simulink model "New_simulation_compare_test"  (R2018b)
settings: Solver=VariableStepAuto  StartTime=0.0  StopTime=10.0  RelTol=1e-3
undefined symbols (not defined in the file or in its folder): DiscIntNeverNeededParam, sigbuilder_block
libraries: commchan3 x2, simulink x2, visionstatistics x1
settings Model: Creator=UWEcocar  LastModifiedBy=UWEcocar

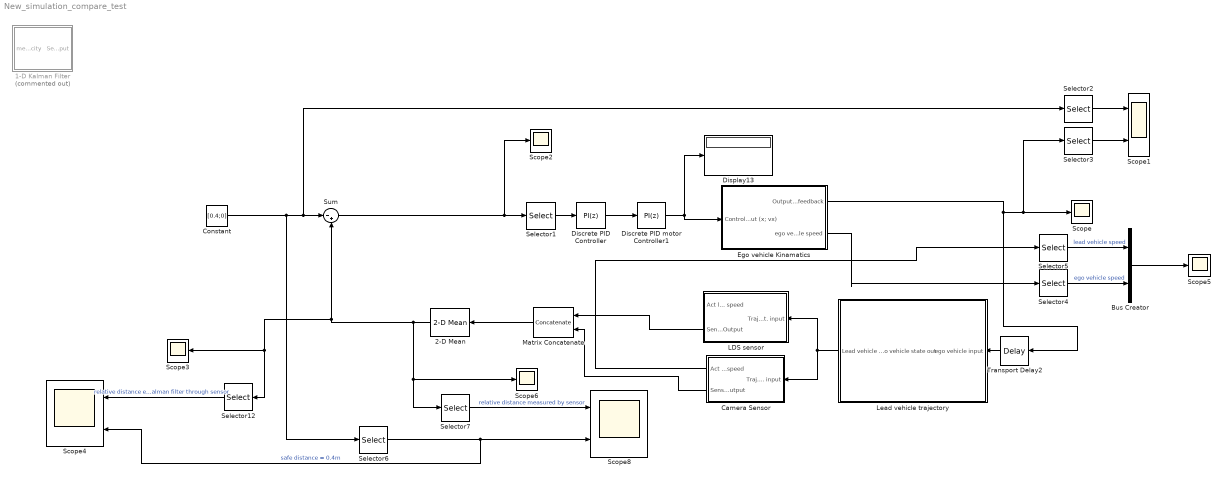
== system New_simulation_compare_test ==
  1-D Kalman Filter : Subsystem  Commented=on
  2-D Mean : visionstatistics/2-D Mean  run=off  reset_popup=None  directionMode=Each row  dimension=1  treatSBRowAsCol=on  roiEnable=off  roiType=Rectangles  roiPortion=Entire ROI  roiOutput=Individual statistics for each ROI  roiFlag=off  outputDataTypeStr=Inherit: Same as accumulator  outputLastDataTypeStr=Inherit: Same as accumulator  outputMin=[]  outputMax=[]  accumMode=Binary point scaling  accumWordLength=32  accumFracLength=0  accumDataTypeStr=fixdt([],32,0)  accumLastDataTypeStr=fixdt([],32,0)  roundingMode=Floor  overflowMode=off
      settings: SourceProductName=Computer Vision System Toolbox  SourceProductBaseCode=VP
  Bus Creator : BusCreator  Inputs=2
  Camera Sensor : Subsystem
  Constant : Constant  Value=[0.4;0]  VectorParams1D=off
  Discrete PID Controller : simulink/Continuous/PID Controller  Controller=PI  Form=Parallel  TimeDomain=Discrete-time  SampleTime=-1  IntegratorMethod=Forward Euler  FilterMethod=Forward Euler  ControllerParametersSource=internal  P=.26  I=.001  D=0  UseFilter=on  N=100  TunerSelectOption=Transfer Function Based (PID Tuner App)  InitialConditionSource=internal  InitialConditionForIntegrator=0  InitialConditionForFilter=0  DifferentiatorICPrevScaledInput=0  ExternalReset=none  TrackingMode=off  Kt=1  LimitOutput=on  UpperSaturationLimit=0.2  LowerSaturationLimit=-0.2  LinearizeAsGain=off  AntiWindupMode=clamping  Kb=1  POutMin=[]  POutMax=[]  IOutMin=[]  IOutMax=[]  DOutMin=[]  DOutMax=[]  NOutMin=[]  NOutMax=[]  SumOutMin=[]  SumOutMax=[]  SaturationOutMin=[]  SaturationOutMax=[]  PParamMin=[]  PParamMax=[]  IParamMin=[]  IParamMax=[]  DParamMin=[]  DParamMax=[]  NParamMin=[]  NParamMax=[]  KbParamMin=[]  KbParamMax=[]  KtParamMin=[]  KtParamMax=[]  KbOutMin=[]  KbOutMax=[]  KtOutMin=[]  KtOutMax=[]  IntegratorOutMin=[]  IntegratorOutMax=[]  FilterOutMin=[]  FilterOutMax=[]  SumI1OutMin=[]  SumI1OutMax=[]  SumI2OutMin=[]  SumI2OutMax=[]  SumI3OutMin=[]  SumI3OutMax=[]  SumI4OutMin=[]  SumI4OutMax=[]  SumDOutMin=[]  SumDOutMax=[]  DifferentiatorOutMin=[]  DifferentiatorOutMax=[]  FilterDiffOutCoefMin=[]  FilterDiffOutCoefMax=[]  ReciprocalOutMin=[]  ReciprocalOutMax=[]  SumDenOutMin=[]  SumDenOutMax=[]  SumNumOutMin=[]  SumNumOutMax=[]  DivideOutMin=[]  DivideOutMax=[]  IntegratorContinuousStateAttributes=''  IntegratorStateMustResolveToSignalObject=off  IntegratorRTWStateStorageClass=Auto  FilterContinuousStateAttributes=''  FilterStateMustResolveToSignalObject=off  FilterRTWStateStorageClass=Auto  ParallelPVariant=InternalParameters  IdealPVariant=Disabled  IVariant=InternalParameters  DVariant=Disabled  IntegratorVariant=Discrete  SatVariant=Enabled  AWVariant=DiscClampingParallel  PCopyVariant=Disabled  TRVariant=Disabled  FdbkBlocksVariant=Forward  IdealPFdbkVariant=Disabled  SatFdbkVariant=Disabled  DerivativeFilterVariant=Disabled  NVariant=Disabled  NCopyVariant=Disabled_SignalSpec  FilterICVariant=Disabled  IntegratorICVariant=InternalICs  ExternalResetVariant=Disabled  TRSumVariant=Passthrough  SumFdbkVariant=Disabled  SumVariant=Sum_PI
  Discrete PID motor Controller1 : simulink/Continuous/PID Controller  Controller=PI  Form=Parallel  TimeDomain=Discrete-time  SampleTime=-1  IntegratorMethod=Forward Euler  FilterMethod=Forward Euler  ControllerParametersSource=internal  P=0.7813  I=0.0153  D=0  UseFilter=on  N=100  TunerSelectOption=Transfer Function Based (PID Tuner App)  InitialConditionSource=internal  InitialConditionForIntegrator=0  InitialConditionForFilter=0  DifferentiatorICPrevScaledInput=0  ExternalReset=none  TrackingMode=off  Kt=1  LimitOutput=on  UpperSaturationLimit=0.2  LowerSaturationLimit=-0.2  LinearizeAsGain=off  AntiWindupMode=clamping  Kb=1  POutMin=[]  POutMax=[]  IOutMin=[]  IOutMax=[]  DOutMin=[]  DOutMax=[]  NOutMin=[]  NOutMax=[]  SumOutMin=[]  SumOutMax=[]  SaturationOutMin=[]  SaturationOutMax=[]  PParamMin=[]  PParamMax=[]  IParamMin=[]  IParamMax=[]  DParamMin=[]  DParamMax=[]  NParamMin=[]  NParamMax=[]  KbParamMin=[]  KbParamMax=[]  KtParamMin=[]  KtParamMax=[]  KbOutMin=[]  KbOutMax=[]  KtOutMin=[]  KtOutMax=[]  IntegratorOutMin=[]  IntegratorOutMax=[]  FilterOutMin=[]  FilterOutMax=[]  SumI1OutMin=[]  SumI1OutMax=[]  SumI2OutMin=[]  SumI2OutMax=[]  SumI3OutMin=[]  SumI3OutMax=[]  SumI4OutMin=[]  SumI4OutMax=[]  SumDOutMin=[]  SumDOutMax=[]  DifferentiatorOutMin=[]  DifferentiatorOutMax=[]  FilterDiffOutCoefMin=[]  FilterDiffOutCoefMax=[]  ReciprocalOutMin=[]  ReciprocalOutMax=[]  SumDenOutMin=[]  SumDenOutMax=[]  SumNumOutMin=[]  SumNumOutMax=[]  DivideOutMin=[]  DivideOutMax=[]  IntegratorContinuousStateAttributes=''  IntegratorStateMustResolveToSignalObject=off  IntegratorRTWStateStorageClass=Auto  FilterContinuousStateAttributes=''  FilterStateMustResolveToSignalObject=off  FilterRTWStateStorageClass=Auto  ParallelPVariant=InternalParameters  IdealPVariant=Disabled  IVariant=InternalParameters  DVariant=Disabled  IntegratorVariant=Discrete  SatVariant=Enabled  AWVariant=DiscClampingParallel  PCopyVariant=Disabled  TRVariant=Disabled  FdbkBlocksVariant=Forward  IdealPFdbkVariant=Disabled  SatFdbkVariant=Disabled  DerivativeFilterVariant=Disabled  NVariant=Disabled  NCopyVariant=Disabled_SignalSpec  FilterICVariant=Disabled  IntegratorICVariant=InternalICs  ExternalResetVariant=Disabled  TRSumVariant=Passthrough  SumFdbkVariant=Disabled  SumVariant=Sum_PI
  Display13 : Display
  Ego vehicle Kinamatics : Subsystem
  LDS sensor : Subsystem
  Lead vehicle trajectory : Subsystem
  Matrix Concatenate : Concatenate  Mode=Multidimensional array  ConcatenateDimension=2
  Scope{,2..3,5..6} (5 alike) : Scope
  Scope1 : Scope  NumInputPorts=2
  Scope4 : Scope  NumInputPorts=2
  Scope8 : Scope  NumInputPorts=2
  Selector{1..4,6..7,12} (7 alike) : Selector  InputPortWidth=2  IndexOptions=Index vector (dialog)  Indices=[1]  OutputSizes=1
  Selector5 : Selector  InputPortWidth=2  IndexOptions=Index vector (dialog)  Indices=[2]  OutputSizes=1
  Sum : Sum  Inputs=|-+
  Transport Delay2 : TransportDelay  DelayTime=0.8
  wires:
  LDS sensor/2(Sensor Output) -> Matrix Concatenate/1
  Selector12/1 -> Scope4/1  "relative distance estimated be kalman filter through sensor"
  Selector4/1 -> Bus Creator/2  "ego vehicle speed"
  Selector2/1 -> Scope1/1
  Selector6/1 -> Scope4/2, Scope8/2  "safe distance = 0.4m"
  Transport Delay2/1 -> Lead vehicle trajectory/1(ego vehicle input)
  Selector5/1 -> Bus Creator/1  "lead vehicle speed"
  Discrete PID motor Controller1/1 -> Display13/1, Ego vehicle Kinamatics/1(Controller input (x; vx))
  Discrete PID Controller/1 -> Discrete PID motor Controller1/1
  Sum/1 -> Scope2/1, Selector1/1
  Camera Sensor/2(Sensor Output) -> Matrix Concatenate/2
  2-D Mean/1 -> Sum/2, Scope3/1, Selector12/1, Scope6/1, Selector7/1
  Selector1/1 -> Discrete PID Controller/1
  Ego vehicle Kinamatics/2(ego vehicle speed) -> Selector4/1
  Selector7/1 -> Scope8/1  "relative distance measured by sensor"
  Matrix Concatenate/1 -> 2-D Mean/1
  Bus Creator/1 -> Scope5/1
  Selector3/1 -> Scope1/2
  Constant/1 -> Selector6/1, Selector2/1, Sum/1
  Ego vehicle Kinamatics/1(Output for sensor feedback) -> Transport Delay2/1, Selector3/1, Scope/1
  Camera Sensor/1(Act lead vehicle speed) -> Selector5/1
  Lead vehicle trajectory/1(Lead vehicle traject. and ego vehicle state out) -> LDS sensor/1(Traject. input), Camera Sensor/1(Traject. input)

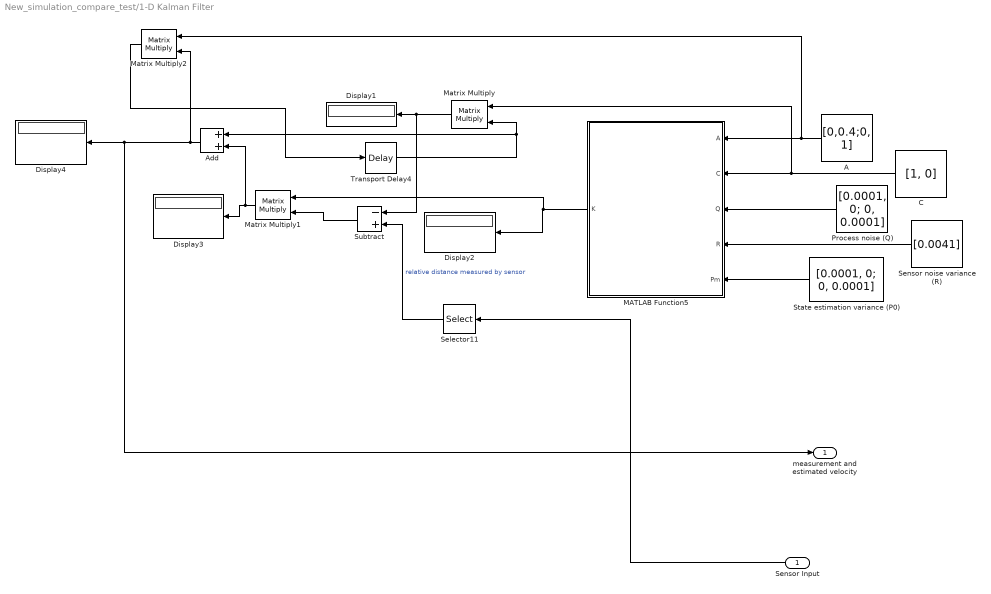
== system New_simulation_compare_test/1-D Kalman Filter ==
  Sensor Input : Inport
  A : Constant  Value=[0,0.4;0, 1]  VectorParams1D=off
  Add : Sum
  C : Constant  Value=[1, 0]  VectorParams1D=off
  Display{1..4} (4 alike) : Display
  MATLAB Function5 : MATLAB Function  TreatAsAtomicUnit=on
  Matrix Multiply : Product  Multiplication=Matrix(*)
  Matrix Multiply1 : Product  Multiplication=Matrix(*)
  Matrix Multiply2 : Product  Multiplication=Matrix(*)
  Process noise (Q) : Constant  Value=|  VectorParams1D=off
      | [0.0001, 0;
      | 0, 0.0001]
  Selector11 : Selector  InputPortWidth=2  IndexOptions=Index vector (dialog)  Indices=[1]  OutputSizes=1
  Sensor noise variance (R) : Constant  Value=[0.0041]  VectorParams1D=off
  State estimation variance (P0) : Constant  Value=[0.0001, 0; 0, 0.0001]  VectorParams1D=off
  Subtract : Sum  Inputs=-+
  Transport Delay4 : TransportDelay  DelayTime=0.4
  measurement and estimated velocity : Outport
  wires:
  MATLAB Function5/1(K) -> Matrix Multiply1/1, Display2/1
  Matrix Multiply1/1 -> Add/2, Display3/1
  Selector11/1 -> Subtract/2  "relative distance measured by sensor"
  Matrix Multiply2/1 -> Transport Delay4/1
  A/1 -> Matrix Multiply2/1, MATLAB Function5/1(A)
  State estimation variance (P0)/1 -> MATLAB Function5/5(Pm)
  Add/1 -> Matrix Multiply2/2, measurement and estimated velocity/1, Display4/1
  C/1 -> Matrix Multiply/1, MATLAB Function5/2(C)
  Process noise (Q)/1 -> MATLAB Function5/3(Q)
  Matrix Multiply/1 -> Subtract/1, Display1/1
  Sensor noise variance (R)/1 -> MATLAB Function5/4(R)
  Sensor Input/1 -> Selector11/1
  Subtract/1 -> Matrix Multiply1/2
  Transport Delay4/1 -> Add/1, Matrix Multiply/2

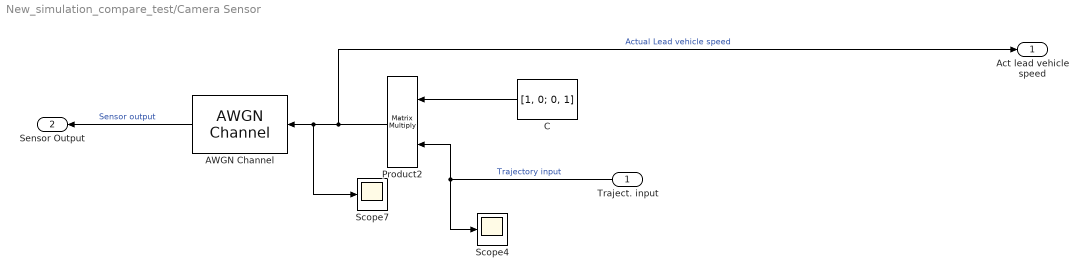
== system New_simulation_compare_test/Camera Sensor ==
  Traject. input : Inport
  AWGN Channel : commchan3/AWGN Channel  InputProcessing=Columns as channels (frame based)  seed=67  noiseMode="Signal to noise ratio  (SNR)"  EbNodB=100  EsNodB=10  SNRdB=19  bitsPerSym=1  Ps=1  Tsym=0.4  variance=1
  C : Constant  Value="[1, 0;    0, 1]"  VectorParams1D=off
  Product2 : Product  Multiplication=Matrix(*)
  Scope4 : Scope
  Scope7 : Scope
  Act lead vehicle speed : Outport
  Sensor Output : Outport  Port=2
  wires:
  Traject. input/1 -> Product2/2, Scope4/1  "Trajectory input"
  AWGN Channel/1 -> Sensor Output/1  "Sensor output"
  C/1 -> Product2/1
  Product2/1 -> Act lead vehicle speed/1, AWGN Channel/1, Scope7/1  "Actual Lead vehicle speed"

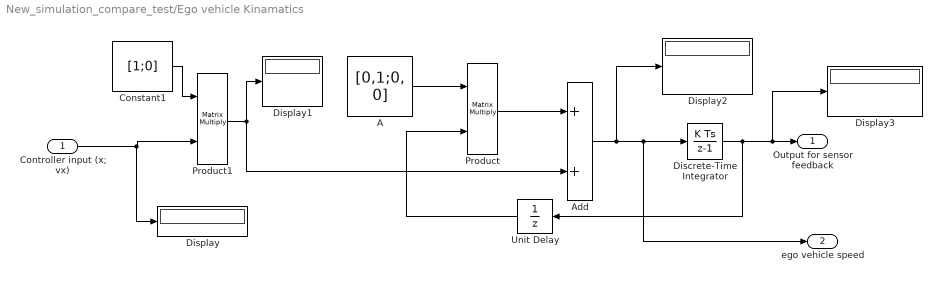
== system New_simulation_compare_test/Ego vehicle Kinamatics ==
  Controller input (x; vx) : Inport
  A : Constant  Value=[0,1;0, 0]  VectorParams1D=off
  Add : Sum
  Constant1 : Constant  Value=[1;0]  VectorParams1D=off
  Discrete-Time Integrator : DiscreteIntegrator  InitialCondition=[0;0]  SampleTime=-1  ICPrevOutput=DiscIntNeverNeededParam  ICPrevScaledInput=DiscIntNeverNeededParam
  Display{,1..3} (4 alike) : Display
  Product : Product  Multiplication=Matrix(*)
  Product1 : Product  Multiplication=Matrix(*)
  Unit Delay : UnitDelay  SampleTime=-1
  Output for sensor feedback : Outport
  ego vehicle speed : Outport  Port=2
  wires:
  Discrete-Time Integrator/1 -> Unit Delay/1, Display3/1, Output for sensor feedback/1
  A/1 -> Product/1
  Controller input (x; vx)/1 -> Display/1, Product1/2
  Product1/1 -> Display1/1, Add/2
  Add/1 -> Display2/1, ego vehicle speed/1, Discrete-Time Integrator/1
  Product/1 -> Add/1
  Constant1/1 -> Product1/1
  Unit Delay/1 -> Product/2

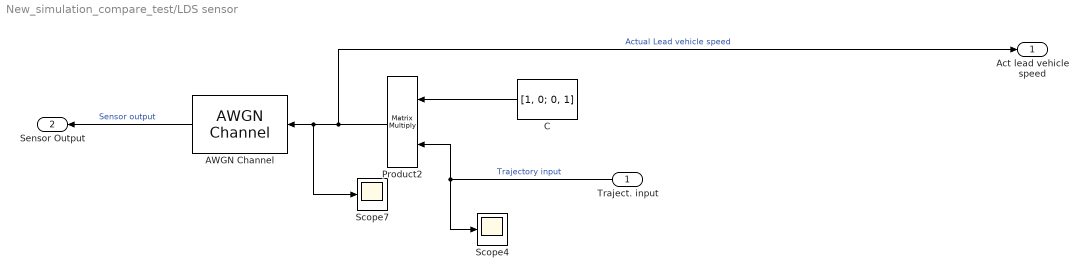
== system New_simulation_compare_test/LDS sensor ==
  Traject. input : Inport
  AWGN Channel : commchan3/AWGN Channel  InputProcessing=Columns as channels (frame based)  seed=67  noiseMode="Signal to noise ratio  (SNR)"  EbNodB=100  EsNodB=10  SNRdB=27  bitsPerSym=1  Ps=1  Tsym=0.4  variance=1
  C : Constant  Value="[1, 0;    0, 1]"  VectorParams1D=off
  Product2 : Product  Multiplication=Matrix(*)
  Scope4 : Scope
  Scope7 : Scope
  Act lead vehicle speed : Outport
  Sensor Output : Outport  Port=2
  wires:
  Product2/1 -> Act lead vehicle speed/1, AWGN Channel/1, Scope7/1  "Actual Lead vehicle speed"
  C/1 -> Product2/1
  Traject. input/1 -> Product2/2, Scope4/1  "Trajectory input"
  AWGN Channel/1 -> Sensor Output/1  "Sensor output"

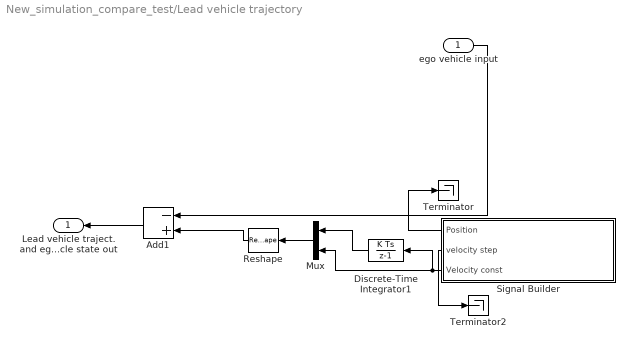
== system New_simulation_compare_test/Lead vehicle trajectory ==
  ego vehicle input : Inport
  Add1 : Sum  Inputs=-+
  Discrete-Time Integrator1 : DiscreteIntegrator  InitialCondition=0.6  SampleTime=-1  ICPrevOutput=DiscIntNeverNeededParam  ICPrevScaledInput=DiscIntNeverNeededParam
  Mux : Mux  Inputs=2
  Reshape : Reshape  OutputDimensionality=Column vector (2-D)
  Signal Builder : Subsystem  Tag=STV Subsys  LoadFcn=sigbuilder_block('load');  StartFcn=sigbuilder_block('start');  StopFcn=sigbuilder_block('stop');  ClipboardFcn=sigbuilder_block('clipboard');  mask(Sigbuilder block){tuvar=[0:10]}
      mask help: Simulink:masks:SigbuilderBlock_MD
      mask init:
      | if ~strcmp(get_param(bdroot(gcbh),'SimulationStatus'),'stopped') tuvar = sigbuilder_block('maskInit'); end
      settings: CopyFcn=sigbuilder_block('copy');  DeleteFcn=sigbuilder_block('delete');  ModelCloseFcn=sigbuilder_block('modelClose');  PreSaveFcn=sigbuilder_block('preSave');  PauseFcn=sigbuilder_block('pause');  ContinueFcn=sigbuilder_block('continue');  NameChangeFcn=sigbuilder_block('namechange');  OpenFcn=sigbuilder_block('open',[439.5 191.25 550.5 399.75 ]);  CloseFcn=sigbuilder_block('close');
      mask Display: plot(0, 0, 100, 100,[2, 2, 32, 32, 2], [68, 8, 8, 68, 68],[32, 2], [38, 38], [32, 19, 2],[53, 60, 44], [32, 17, 17, 2],[16, 16, 31, 31]);txt = getActiveGroup(gcbh);text(2, 100, txt,'verticalAlignment', 'top');
  Terminator : Terminator
  Terminator2 : Terminator
  Lead vehicle traject. and ego vehicle state out : Outport
  wires:
  Signal Builder/1(Position) -> Terminator/1
  Mux/1 -> Reshape/1
  Reshape/1 -> Add1/2
  Discrete-Time Integrator1/1 -> Mux/1
  ego vehicle input/1 -> Add1/1
  Add1/1 -> Lead vehicle traject. and ego vehicle state out/1
  Signal Builder/3(Velocity const) -> Mux/2, Discrete-Time Integrator1/1
  Signal Builder/2(velocity step) -> Terminator2/1

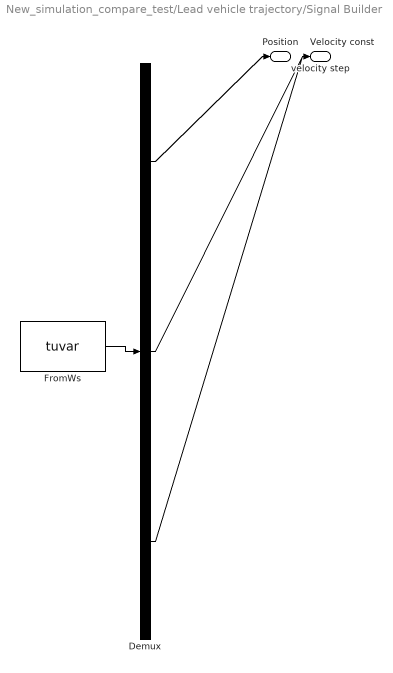
== system New_simulation_compare_test/Lead vehicle trajectory/Signal Builder ==
  Demux : Demux  Tag=STV Demux  Outputs=3
  FromWs : FromWorkspace  Tag=STV FromWs  VariableName=tuvar  SampleTime=0
      SigBuilderData=|
      | common.afterFinalStr = 'Extrapolate'
      | common.sampleTime = 0
      | dataSet.timeRange = [0 120]
      | dataSet.name = 'Group 1'
      | sbobj.Groups.Name = 'Group 1'
      | sbobj.Groups.Signals(1).Name = 'Position'
      | sbobj.Groups.Signals(1).XData = [0 6 10 120]
      | sbobj.Groups.Signals(1).YData = [0 0.705 1 1]
      | sbobj.Groups.Signals(2).Name = 'velocity step'
      | sbobj.Groups.Signals(2).XData = [0 60 60 120]
      | sbobj.Groups.Signals(2).YData = [0.1 0.1 0.2 0.2]
      | sbobj.Groups.Signals(3).Name = 'Velocity const'
      | sbobj.Groups.Signals(3).XData = [0 60 120]
      | sbobj.Groups.Signals(3).YData = [0.07 0.07 0.07]
      | sbobj.Groups.TimeRange = [0 120]
  Position : Outport  Tag=STV Outport
  velocity step : Outport  Tag=STV Outport  Port=2
  Velocity const : Outport  Tag=STV Outport  Port=3
  wires:
  FromWs/1 -> Demux/1
  Demux/1 -> Position/1
  Demux/2 -> velocity step/1
  Demux/3 -> Velocity const/1

== matlab function New_simulation_compare_test/1-D Kalman Filter/MATLAB Function5 ==
  data: A input; K output; C input; Q input; R input; Pm input
% This code has referred from
% https://www.cs.cmu.edu/~cga/dynopt/kalman/kalman.html and
% https://statweb.stanford.edu/~candes/acm116/Handouts/Kalman.pdf
% for more info check it out.
% as we are having longitudinal autonomy, therefore taking simple state transition matrix!!
function K  = sim_vel_est_kalman_filt_1D(A, C, Q, R, Pm)
%{
    C = [1, 0];
R = [0.000225];
Q = [0.0001, 0;
      0, 0.0001];
P0 = [0.0001, 0;
       0, 0.0001];
    
sem = [0, 0]';
          if detectionClusters{1, 1}.Measurement(1, :) >= 0.5
            Q = [(0.035 * detectionClusters{1, 1}.Measurement(1, :))^2, 0;
                    0,  (0.035 * detectionClusters{1, 1}.Measurement(1, :))^2];
          end
          if detectionClusters{1, 1}.Measurement(1, :) >= 0.5
                R = [(0.05*detectionClusters{1, 1}.Measurement(1, :))^2];
          end
          if detectionClusters{1, 1}.Measurement(1, :) >= 0.5
                P0 = [(0.035 * detectionClusters{1, 1}.Measurement(1, :))^2, 0;
                        0 , (0.035 * detectionClusters{1, 1}.Measurement(1, :))^2];
          end
          dt = toc(tStart);
          tStart = tic;
          A = [1, dt;
                0, 1];
%}
% designing the Kalman filter

for i = 1:1000
% measurement step

    S = C * Pm * C' + R;
    %K = Pm*C'*inv(S); % change this inverse thing to solve with solutions of linear equations.
    % changing to linear eq solution:
    K =  Pm*C' * inv(S); % as it is 1 D dividing it, but for matrix linsolve is the best to get the "K".

    Pp = Pm - K*C*Pm;
 % prediction step
    Pm = A*Pp*A' + Q;
end

 
end
